simulink model "robot2D_2018"  (Simulink 9.2)
settings: Solver=FixedStepAuto  StartTime=0.0  StopTime=10.0  FixedStep=0.001  RelTol=1e-3
values from neighbouring files (symbols this model uses):
  Kd1 = 2 * zeta * wn * D_diag_const(1,1) - C_diag_const(1,1)    [script.m]
  Kd2 = 2 * zeta * wn * D_diag_const(2,2) - C_diag_const(2,2)    [script.m]
  Kp1 = D_diag_const(1,1) * wn^2    [script.m]
  Kp2 = D_diag_const(2,2) * wn^2    [script.m]
  q1 = 3    [script.m]
  q2 = 3    [script.m]
settings Model: Creator=alexa  LastModifiedBy=UTCN-C12
settings DataIOCC: LimitDataPoints=off  SaveFormat=Dataset  SignalLoggingSaveFormat=Dataset  ReturnWorkspaceOutputs=on
settings OptimizationCC: LifeSpan=auto
settings DebuggingCC: UnderspecifiedInitializationDetection=Simplified  MergeDetectMultiDrivingBlocksExec=error  FcnCallInpInsideContextMsg=error  UnconnectedInputMsg=none  UnconnectedOutputMsg=none  UnconnectedLineMsg=none  StateNameClashWarn=none  SFUnexpectedBacktrackingDiag=error  SFNoUnconditionalDefaultTransitionDiag=error  SFExecutionAtInitializationDiag=warning  SFMachineParentedDataDiag=error
settings HardwareCC: ProdBitPerPointer=64  ProdBitPerSizeT=64  ProdBitPerPtrDiffT=64  ProdLargestAtomicFloat=Float  ProdIntDivRoundTo=Zero  ProdEndianess=LittleEndian  ProdWordSize=64  ProdHWDeviceType=Intel->x86-64 (Windows64)
settings ModelReferenceCC: PropagateSignalLabelsOutOfModel=on
settings SFSimCC: SimUseLocalCustomCode=on
settings RTWCC: RTWUseLocalCustomCode=on
settings CodeAppCC: StateflowObjectComments=off
settings GRTTargetCC: TargetLangStandard=C99 (ISO)  GeneratePreprocessorConditionals=Use local settings  CombineOutputUpdateFcns=on  GRTInterface=off
settings ConfigComp: CovMetricSettings=dwe  CovHtmlReporting=off  CovSaveCumulativeToWorkspaceVar=off  CovSaveSingleToWorkspaceVar=off  CovExternalEMLEnable=on

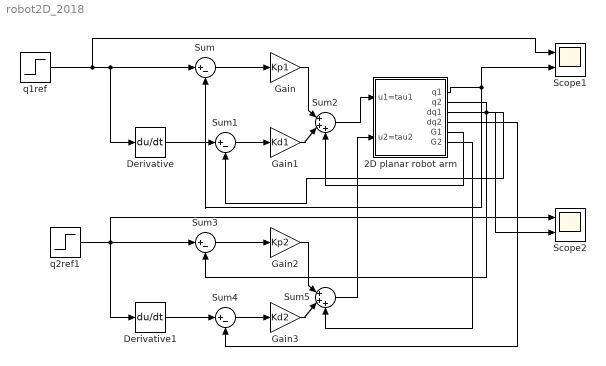
== system robot2D_2018 ==
  2D planar robot arm : Subsystem
  Derivative : Derivative
  Derivative1 : Derivative
  Gain : Gain  Gain=Kp1
  Gain1 : Gain  Gain=Kd1
  Gain2 : Gain  Gain=Kp2
  Gain3 : Gain  Gain=Kd2
  Scope1 : Scope  NumInputPorts=2
  Scope2 : Scope  NumInputPorts=2
  Sum{,1,3..4} (4 alike) : Sum  Inputs=|+-
  Sum2 : Sum  Inputs=|+++
  Sum5 : Sum  Inputs=|+++
  q1ref : Step  Before=q1  After=q1  SampleTime=0
  q2ref1 : Step  Before=q2  After=q2  SampleTime=q2
  wires:
  2D planar robot arm/3(dq1) -> Sum1/2
  q1ref/1 -> Scope1/1, Derivative/1, Sum/1
  Sum/1 -> Gain/1
  Derivative/1 -> Sum1/1
  Gain/1 -> Sum2/1
  Sum1/1 -> Gain1/1
  Gain1/1 -> Sum2/2
  Sum2/1 -> 2D planar robot arm/1(u1=tau1)
  Derivative1/1 -> Sum4/1
  Gain3/1 -> Sum5/2
  Gain2/1 -> Sum5/1
  q2ref1/1 -> Derivative1/1, Sum3/1, Scope2/1
  Sum4/1 -> Gain3/1
  Sum3/1 -> Gain2/1
  Sum5/1 -> 2D planar robot arm/2(u2=tau2)
  2D planar robot arm/1(q1) -> Sum/2, Scope1/2
  2D planar robot arm/2(q2) -> Sum3/2, Scope2/2
  2D planar robot arm/5(G1) -> Sum2/3
  2D planar robot arm/6("G2 ") -> Sum5/3
  2D planar robot arm/4(dq2) -> Sum4/2

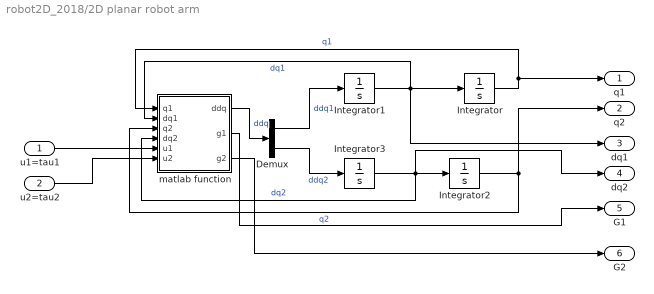
== system robot2D_2018/2D planar robot arm ==
  u1=tau1 : Inport
  u2=tau2 : Inport  Port=2
  Demux : Demux  Outputs=2
  Integrator{,1..3} (4 alike) : Integrator
  matlab function : MATLAB Function  TreatAsAtomicUnit=on
  q1 : Outport  VectorParamsAs1DForOutWhenUnconnected=on
  q2 : Outport  Port=2  VectorParamsAs1DForOutWhenUnconnected=on
  dq1 : Outport  Port=3  VectorParamsAs1DForOutWhenUnconnected=on
  dq2 : Outport  Port=4  VectorParamsAs1DForOutWhenUnconnected=on
  G1 : Outport  Port=5  VectorParamsAs1DForOutWhenUnconnected=on
  "G2 " : Outport  Port=6  VectorParamsAs1DForOutWhenUnconnected=on
  wires:
  u1=tau1/1 -> matlab function/5(u1)
  Integrator1/1 -> dq1/1, matlab function/2(dq1), Integrator/1  "dq1"
  Demux/2 -> Integrator3/1  "ddq2"
  Integrator2/1 -> q2/1, matlab function/3(q2)  "q2"
  Integrator3/1 -> dq2/1, matlab function/4(dq2), Integrator2/1  "dq2"
  matlab function/1(ddq) -> Demux/1  "ddq"
  u2=tau2/1 -> matlab function/6(u2)
  Demux/1 -> Integrator1/1  "ddq1"
  Integrator/1 -> q1/1, matlab function/1(q1)  "q1"
  matlab function/2(g1) -> G1/1
  matlab function/3(g2) -> "G2 "/1

== matlab function 2D planar robot arm/matlab function ==
  data: q1 input double; ddq output double; dq1 input double; q2 input double; dq2 input double; u1 input double; u2 input double; g1 output double; g2 output double
function [ddq,g1,g2] = fcn(q1,dq1,q2,dq2,u1,u2)


D=[0.003515*cos(q2) + 0.000925*cos(q2)^2 + 0.026254,        0
                                               0, 0.023625];
C=[0.24 - 0.0017575*dq2*sin(q2) - 0.0004625*dq2*sin(2.0*q2), - 0.0004625*dq1*sin(2.0*q2) - 0.0017575*dq1*sin(q2)
       0.0004625*dq1*sin(2.0*q2) + 0.0017575*dq1*sin(q2),                                                0.16];
G=[0.30055*sin(q1) - 0.18149*cos(q2)*sin(q1);
                 -0.18149*cos(q1)*sin(q2)];

F_prim =[0;0]
g1=G(1);
g2=G(2);


ddq=inv(D)*(-C*[dq1;dq2]-G+[u1;u2]-F_prim);
